simulink model "board_unspecific_TLC5952"  (R2016b)
settings: Solver=FixedStepDiscrete  StartTime=0.0  StopTime=10.0  FixedStep=1e-3  RelTol=1e-3
settings Model: Creator=oh  LastModifiedBy=oh
settings OptimizationCC: DefaultParameterBehavior=Inlined
settings DebuggingCC: ParameterTunabilityLossMsg=error
settings HardwareCC: ProdBitPerPointer=32  ProdBitPerSizeT=32  ProdBitPerPtrDiffT=32  ProdLargestAtomicInteger=Long  ProdLargestAtomicFloat=Double  ProdWordSize=32  ProdHWDeviceType=ARM Compatible->ARM Cortex
settings RTWCC: SystemTargetFile=mbed.tlc  TemplateMakefile=mbed.tmf  Description=Mbed Target (Embedded Target)  GenerateReport=on  IncludeHyperlinkInReport=on  LaunchReport=on  TargetLang=C++  GenerateTraceInfo=on  GenerateTraceReport=on  GenerateTraceReportSl=on  GenerateTraceReportSf=on  GenerateTraceReportEml=on
settings CodeAppCC: ForceParamTrailComments=on  IgnoreCustomStorageClasses=off  OperatorAnnotations=on  SimulinkDataObjDesc=on  SFDataObjDesc=on  MATLABFcnDesc=on  InsertBlockDesc=on  MATLABSourceComments=on
settings STFCustomTargetCC: TargetLibSuffix=.a  TargetLangStandard=C++03 (ISO)  GenerateSampleERTMain=on  CombineOutputUpdateFcns=on  ERTCustomFileBanners=on  SupportContinuousTime=off  SupportNonInlinedSFcns=off  RemoveResetFunc=on  MATLABClassNameForMDSCustomization=Simulink.SoftwareTarget.ERTCustomization  GRTInterface=off  SystemTargetFile=mbed.tlc
settings ERTTargetCC: TargetLangStandard=C++03 (ISO)  GenerateSampleERTMain=on  ParMdlRefBuildCompliant=off  CompOptLevelCompliant=off  ConcurrentExecutionCompliant=off  ERTFirstTimeCompliant=off  ModelStepFunctionPrototypeControlCompliant=off  CPPClassGenCompliant=off  UseToolchainInfoCompliant=off  InlinedParameterPlacement=NonHierarchical  ERTCustomFileTemplate=mbed_file_process.tlc

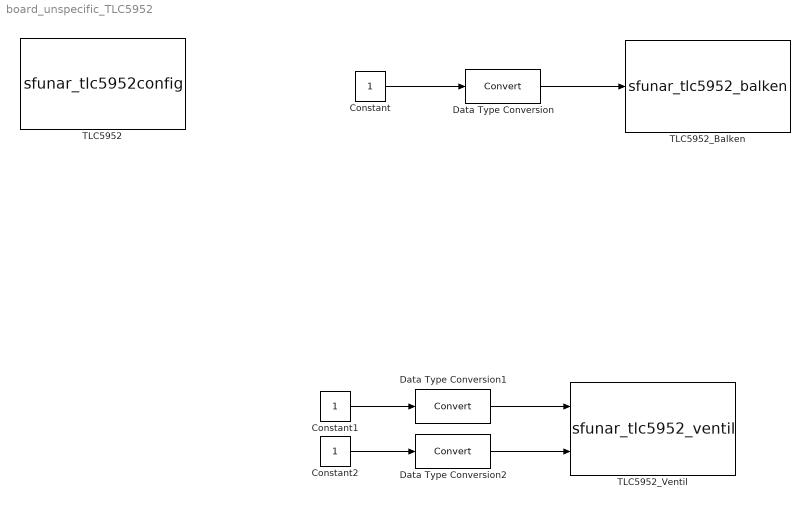
== system board_unspecific_TLC5952 ==
  Constant : Constant
  Constant1 : Constant
  Constant2 : Constant
  Data Type Conversion : DataTypeConversion
  Data Type Conversion1 : DataTypeConversion
  Data Type Conversion2 : DataTypeConversion
  TLC5952 : S-Function  Priority=0  FunctionName=sfunar_tlc5952config  Parameters=uint8(P1),uint8(P2),uint8(P3),uint8(P4),uint8(P5),uint8(P6),uint8(P7),uint8(P8),uint8(P9),uint8(P10)  SFunctionDeploymentMode=off  EnableBusSupport=off  mask(TLC5952 Configuration){P1=B, P2=12, P3=B, P4=13, P5=B, P6=14, P7=B, P8=15, P9=10, P10=0}
      mask prompts: P1 "Clock Port:"; P2 "Pin Number (1-16):"; P3 "Data Port:"; P4 "Pin Number (1-16):"; P5 "Latch Port:"; P6 "Pin Number (1-16):"; P7 "Blank Port:"; P8 "Pin Number (1-16):"; P9 "LED Strom(0-15): [mA]"; P10 "TLC5952 Nummer(0-5):"
      mask help: Config für alle Pins des TLC5952 und den Strom
      mask Help: helpview([mbed_getTargetRootPath '/doc/_build/htmlhelp/chapters/I2c_Config_en.html'])
      mask TypeOptions P1: A | B | C | D | E | F
      mask TypeOptions P2: 0 | 1 | 2 | 3 | 4 | 5 | 6 | 7 | 8 | 9 | 10 | 11 | 12 | 13 | 14 | 15
      mask TypeOptions P3: A | B | C | D | E | F
      mask TypeOptions P4: 0 | 1 | 2 | 3 | 4 | 5 | 6 | 7 | 8 | 9 | 10 | 11 | 12 | 13 | 14 | 15
      mask TypeOptions P5: A | B | C | D | E | F
      mask TypeOptions P6: 0 | 1 | 2 | 3 | 4 | 5 | 6 | 7 | 8 | 9 | 10 | 11 | 12 | 13 | 14 | 15
      mask TypeOptions P7: A | B | C | D | E | F
      mask TypeOptions P8: 0 | 1 | 2 | 3 | 4 | 5 | 6 | 7 | 8 | 9 | 10 | 11 | 12 | 13 | 14 | 15
      mask TypeOptions P10: 0 | 1 | 2 | 3 | 4
      mask Display:
      | disp([' Clock: ' P1+64 '.' num2str(P2-1)]);
      | disp([' Data: ' P3+64, '.' num2str(P4-1) '\n\n']);
      | disp([' Latch: ' P5+64, '.' num2str(P6-1) '\n\n\n\n']);
      | disp(['\n\n Blank: ' P7+64, '.' num2str(P8-1)]);
      | disp(['\n\n\n\n Strom: ' num2str(P9) ' mA']);
      | disp(['TLC5952 Nummer ' num2str(P10-1) '\n\n\n\n\n\n' ]);
  TLC5952_Balken : S-Function  Priority=0  FunctionName=sfunar_tlc5952_balken  Parameters=SampleTime,boolean(up_down) ,uint8(P1)  SFunctionDeploymentMode=off  EnableBusSupport=off  mask(TLC5952 Balken){P1=0, up_down=off, SampleTime=-1}
      mask prompts: P1 "TLC5952 Nummer(0-5):"; up_down "Laufrichtung (checked up/ not checked down)"; SampleTime "Sample time (-1 for inherited):"
      mask help: LED Balken mit Richtungseinstellung
      mask Help: helpview([mbed_getTargetRootPath '/doc/_build/htmlhelp/chapters/I2c_Config_en.html'])
      mask TypeOptions P1: 0 | 1 | 2 | 3 | 4
      mask Display:
      | disp(['Balken\n' 'TLC5952 Nummer ' num2str(P1)-1 ]);
      | port_label('input', 1, 'data');
  TLC5952_Ventil : S-Function  Priority=0  FunctionName=sfunar_tlc5952_ventil  Parameters=SampleTime, uint8(P1),uint8(P2)  SFunctionDeploymentMode=off  EnableBusSupport=off  mask(TLC5952 Ventil 6 LED's){P1=0, P2=0, SampleTime=-1}
      mask prompts: P1 "TLC5952 Nummer(0-5):"; P2 "Ventil Nummer(0-3):"; SampleTime "Sample time (-1 for inherited):"
      mask help: Ventil Lauflicht
      mask Help: helpview([mbed_getTargetRootPath '/doc/_build/htmlhelp/chapters/I2c_Config_en.html'])
      mask TypeOptions P1: 0 | 1 | 2 | 3 | 4
      mask TypeOptions P2: 0 | 1 | 2 | 3
      mask Display:
      | disp(['Ventil\n' 'TLC5952 Nummer ' num2str(P1-1) '\nVentil Nummer ' num2str(P2-1) ]);
      | port_label('input', 1, 'an/aus');
      | port_label('input', 2, 'Teiler Sample Time');
  wires:
  Constant/1 -> Data Type Conversion/1
  Constant1/1 -> Data Type Conversion1/1
  Constant2/1 -> Data Type Conversion2/1
  Data Type Conversion/1 -> TLC5952_Balken/1
  Data Type Conversion1/1 -> TLC5952_Ventil/1
  Data Type Conversion2/1 -> TLC5952_Ventil/2
